simulink model "PubIfDecisionLM_MDL"  (R2020b)
settings: configuration reference "DspaceConfig" (kept outside this file)
PostLoadFcn:
  | if any(exist('dsrtsu_mdlpostloadfcn', 'file') ~= 0), dsrtsu_mdlpostloadfcn('Execute', bdroot); end
InitFcn:
  | , if any(exist('dsmpb_private', 'file') ~= 0), dsmpb_private('dsmpb_mdlclblib', 'Init', bdroot); end,
undefined symbols (not defined in the file or in its folder): OFM_OBJ_FUSIONTYPE_E, OFM_OBJ_MOVINGSTATE_E, OFM_OBJ_ORIENTATION_E, OFM_OBJ_TYPE_E, P_LM_Cyc, P_LM_EMLHistKapRcdBufSize, P_LM_EMLHistTrajBaseDis, P_LM_EMLHistTrajPNum, P_LM_EMLKapCorrMaxThre, P_LM_EMLMinKapThre, P_LM_EMLPathDisDiffThre, P_LM_EMLQuaFiltPar, P_LM_EMLTurnActKapThre, P_LM_EMLValidQuaThre, P_LM_FntPath1Disgap, P_LM_FntPath1MinDis, P_LM_FntPath1Timegap, P_LM_FntPath2Disgap, P_LM_FntPath2MinDis, P_LM_FntPath2Timegap, P_LM_FntPath3Disgap, P_LM_FntPath3MinDis, P_LM_FntPath3Timegap, P_LM_FusBLParFiltP, P_LM_FusEVDifC2Thre, P_LM_FusEVOPath1AllVSLDisThre, P_LM_FusEVOPath1AllVSLLostNumThre, P_LM_FusEVOPath1AllVSLQuaThre, P_LM_FusEVOPath1OTLFacNLC, P_LM_FusOTLQuaThre, P_LM_FusOTLSW, P_LM_FusParC0Index, P_LM_FusParC1Index, P_LM_FusParC2Index, P_LM_FusParC3Index, P_LM_FusVSLQuaThre, P_LM_FusVSLSW, P_LM_FusVSLValidSteerWheerAngThre, P_LM_FusVSLValidVxvThre, P_LM_LaneWidth, P_LM_OTLBufTPInfoEvaFactor, P_LM_OTLObjNum, P_LM_OTLObjSelectAgeThre, P_LM_OTLObjSelectDxAssessVx, P_LM_OTLObjSelectDxThre, P_LM_OTLObjSelectVxThre, P_LM_OTLObjSelectVyAssessDx, P_LM_OTLObjSelectVyThre, P_LM_OTLTrajPntBaseDis, P_LM_OTLTrajStdThre, P_LM_VSLAvailLineNum, P_LM_VSLBLSDiffThre, P_LM_VSLBLSDisRatio, P_LM_VSLFusBLParFiltP_C1, P_LM_VSLFusBLParFiltP_C2, P_LM_VSLFusBLParFiltP_C3, P_LM_VSLFusBLParFiltP_Quality, P_LM_VSLHistTrajBaseDis, P_LM_VSLHistTrajPNum, P_LM_VSLLCC0diff ... (+18)
libraries: simulink x145, LM_LIB x43
(part 11 of 24)

== system PubIfDecisionLM_MDL/Subsystem2/DIR/DrivingIntentionRecognition1/DIR_TurnDirProbCalc/DIR_TurnRightProbCalc/DIR_TurnRightProbCalcByCurveKap ==
  kapTraj : Inport
  1-D Lookup Table : Lookup_n-D  NumberOfTableDimensions=1  BreakpointsForDimension1=[0.01,0.014,0.018,0.022,0.026]  Table=[0,0.25,0.5,0.75,1]  InternalRulePriority=Speed  RndMeth=Simplest  InputSameDT=on
  Constant : Constant  Value=0.026  OutDataTypeStr=single
  Constant1 : Constant  OutDataTypeStr=single
  Constant2 : Constant  Value=0.01  OutDataTypeStr=single
  Constant3 : Constant  Value=0  OutDataTypeStr=single
  Constant4 : Constant  Value=-1  OutDataTypeStr=single
  Logical Operator : Logic  AllPortsSameDT=off  OutDataTypeStr=boolean
  Product : Product
  Relational Operator : RelationalOperator  OutDataTypeStr=boolean  RndMeth=Simplest
  Relational Operator1 : RelationalOperator  Operator=<  OutDataTypeStr=boolean  RndMeth=Simplest
  Relational Operator2 : RelationalOperator  OutDataTypeStr=boolean  RndMeth=Simplest
  Switch : Switch  Criteria=u2 ~= 0
  Switch1 : Switch  Criteria=u2 ~= 0
  DIR_TurnRightProbByKapTraj : Outport
  wires:
  kapTraj/1 -> Product/1
  Constant4/1 -> Product/2
  1-D Lookup Table/1 -> Switch1/1
  Switch/1 -> DIR_TurnRightProbByKapTraj/1  "LM_DIRTurnRightProbByKapTraj"
  Relational Operator1/1 -> Logical Operator/1
  Product/1 -> Relational Operator/1, Relational Operator1/1, Relational Operator2/1, 1-D Lookup Table/1
  Switch1/1 -> Switch/3
  Relational Operator/1 -> Switch/2
  Relational Operator2/1 -> Logical Operator/2
  Constant3/1 -> Switch1/3
  Constant/1 -> Relational Operator/2, Relational Operator1/2
  Constant1/1 -> Switch/1
  Logical Operator/1 -> Switch1/2
  Constant2/1 -> Relational Operator2/2

== system PubIfDecisionLM_MDL/Subsystem2/DIR/DrivingIntentionRecognition1/DIR_TurnDirProbCalc/DIR_TurnRightProbCalc/DIR_TurnRightProbCalcByPsiDtOpt ==
  PsiDtOpt : Inport
  1-D Lookup Table : Lookup_n-D  NumberOfTableDimensions=1  BreakpointsForDimension1=[0.11,0.15,0.19,0.23]  Table=[0,0.33,0.67,1]  InternalRulePriority=Speed  RndMeth=Simplest  InputSameDT=on
  Constant : Constant  Value=0.23  OutDataTypeStr=single
  Constant1 : Constant  OutDataTypeStr=single
  Constant2 : Constant  Value=0.11  OutDataTypeStr=single
  Constant3 : Constant  Value=0  OutDataTypeStr=single
  Constant4 : Constant  Value=-1  OutDataTypeStr=single
  Logical Operator : Logic  AllPortsSameDT=off  OutDataTypeStr=boolean
  Product : Product
  Relational Operator : RelationalOperator  OutDataTypeStr=boolean  RndMeth=Simplest
  Relational Operator1 : RelationalOperator  Operator=<  OutDataTypeStr=boolean  RndMeth=Simplest
  Relational Operator2 : RelationalOperator  OutDataTypeStr=boolean  RndMeth=Simplest
  Switch : Switch  Criteria=u2 ~= 0
  Switch1 : Switch  Criteria=u2 ~= 0
  DIR_TurnRightProbByPsiDtopt : Outport
  wires:
  Constant4/1 -> Product/2
  PsiDtOpt/1 -> Product/1
  1-D Lookup Table/1 -> Switch1/1
  Switch/1 -> DIR_TurnRightProbByPsiDtopt/1  "LM_DIRTurnRightProbByPsiDtopt"
  Switch1/1 -> Switch/3
  Constant3/1 -> Switch1/3
  Logical Operator/1 -> Switch1/2
  Relational Operator2/1 -> Logical Operator/2
  Relational Operator1/1 -> Logical Operator/1
  Constant2/1 -> Relational Operator2/2
  Constant1/1 -> Switch/1
  Relational Operator/1 -> Switch/2
  Constant/1 -> Relational Operator/2, Relational Operator1/2
  Product/1 -> Relational Operator/1, Relational Operator1/1, Relational Operator2/1, 1-D Lookup Table/1

== system PubIfDecisionLM_MDL/Subsystem2/DIR/DrivingIntentionRecognition1/DIR_TurnDirProbCalc/DIR_TurnRightProbCalc/DIR_TurnRightProbCalcBySteerWheelAng ==
  SteerWheelAngle : Inport
  SteerWheelAngleSign : Inport  Port=2
  1-D Lookup Table : Lookup_n-D  NumberOfTableDimensions=1  BreakpointsForDimension1=[85,90,95,100]  Table=[0,0.33,0.67,1]  InternalRulePriority=Speed  RndMeth=Simplest  InputSameDT=on
  Constant : Constant  Value=100  OutDataTypeStr=single
  Constant1 : Constant  OutDataTypeStr=single
  Constant2 : Constant  Value=85  OutDataTypeStr=single
  Constant3 : Constant  Value=0  OutDataTypeStr=single
  Constant4 : Constant  OutDataTypeStr=uint8
  Logical Operator : Logic  Inputs=3  AllPortsSameDT=off  OutDataTypeStr=boolean
  Logical Operator1 : Logic  AllPortsSameDT=off  OutDataTypeStr=boolean
  Relational Operator : RelationalOperator  OutDataTypeStr=boolean  RndMeth=Simplest
  Relational Operator1 : RelationalOperator  Operator=<  OutDataTypeStr=boolean  RndMeth=Simplest
  Relational Operator2 : RelationalOperator  OutDataTypeStr=boolean  RndMeth=Simplest
  Relational Operator3 : RelationalOperator  Operator===  OutDataTypeStr=boolean  RndMeth=Simplest
  Switch : Switch  Criteria=u2 ~= 0
  Switch1 : Switch  Criteria=u2 ~= 0
  DIR_TurnRightProbBySteerWheelAng : Outport
  wires:
  [SteerRightFlg] -> Logical Operator/3
  Logical Operator1/1 -> Switch/2
  Relational Operator3/1 -> Logical Operator1/1, [SteerRightFlg]
  Constant4/1 -> Relational Operator3/2
  SteerWheelAngleSign/1 -> Relational Operator3/1
  1-D Lookup Table/1 -> Switch1/1
  Switch1/1 -> Switch/3
  Constant3/1 -> Switch1/3
  Constant1/1 -> Switch/1
  Logical Operator/1 -> Switch1/2
  Constant2/1 -> Relational Operator2/2
  Relational Operator/1 -> Logical Operator1/2
  Relational Operator2/1 -> Logical Operator/2
  Constant/1 -> Relational Operator1/2, Relational Operator/2
  Relational Operator1/1 -> Logical Operator/1
  Switch/1 -> DIR_TurnRightProbBySteerWheelAng/1  "LM_DIRTurnRightProbBySteerWheelAng"
  SteerWheelAngle/1 -> Relational Operator/1, Relational Operator1/1, Relational Operator2/1, 1-D Lookup Table/1

== system PubIfDecisionLM_MDL/Subsystem2/DIR/DrivingIntentionRecognition1/DIR_TurnDirProbCalc/DIR_TurnRightProbCalc/DIR_TurnRightProbCalcByTurnLampSts ==
  RightTurnSWSts : Inport
  Constant : Constant  OutDataTypeStr=uint8
  Constant1 : Constant  OutDataTypeStr=single
  Constant2 : Constant  Value=0  OutDataTypeStr=single
  Relational Operator : RelationalOperator  Operator===  OutDataTypeStr=boolean  RndMeth=Simplest
  Switch : Switch  Criteria=u2 ~= 0
  DIR_TurnRightProbByTurnLampSts : Outport
  wires:
  Switch/1 -> DIR_TurnRightProbByTurnLampSts/1  "LM_DIRTurnRightProbByTurnLampSts"
  Constant2/1 -> Switch/3
  Constant1/1 -> Switch/1
  Relational Operator/1 -> Switch/2
  Constant/1 -> Relational Operator/2
  RightTurnSWSts/1 -> Relational Operator/1

== system PubIfDecisionLM_MDL/Subsystem2/DIR/DrivingIntentionRecognition1/DIR_TurnDirProbCalc/DIR_TurnRightProbCalc/DIR_TurnRightProbCalcByVehSpd ==
  vxvRefMs : Inport
  1-D Lookup Table : Lookup_n-D  NumberOfTableDimensions=1  BreakpointsForDimension1=[12,12.5,13,13.5,14]  Table=[1,0.75,0.5,0.25,0]  InternalRulePriority=Speed  RndMeth=Simplest  InputSameDT=on
  Constant : Constant  Value=12  OutDataTypeStr=single
  Constant1 : Constant  OutDataTypeStr=single
  Constant2 : Constant  Value=14  OutDataTypeStr=single
  Constant3 : Constant  Value=0  OutDataTypeStr=single
  Logical Operator : Logic  AllPortsSameDT=off  OutDataTypeStr=boolean
  Relational Operator : RelationalOperator  Operator=<=  OutDataTypeStr=boolean  RndMeth=Simplest
  Relational Operator1 : RelationalOperator  Operator=>  OutDataTypeStr=boolean  RndMeth=Simplest
  Relational Operator2 : RelationalOperator  Operator=<=  OutDataTypeStr=boolean  RndMeth=Simplest
  Switch : Switch  Criteria=u2 ~= 0
  Switch1 : Switch  Criteria=u2 ~= 0
  LM_DIRTurnRightProbByVehSpd : Outport
  wires:
  Switch/1 -> LM_DIRTurnRightProbByVehSpd/1  "LM_DIRTurnRightProbByVehSpd"
  Constant3/1 -> Switch1/3
  1-D Lookup Table/1 -> Switch1/1
  Switch1/1 -> Switch/3
  Logical Operator/1 -> Switch1/2
  Relational Operator2/1 -> Logical Operator/2
  Relational Operator1/1 -> Logical Operator/1
  Constant2/1 -> Relational Operator2/2
  Relational Operator/1 -> Switch/2
  Constant1/1 -> Switch/1
  Constant/1 -> Relational Operator1/2, Relational Operator/2
  vxvRefMs/1 -> Relational Operator/1, 1-D Lookup Table/1, Relational Operator1/1, Relational Operator2/1

== system PubIfDecisionLM_MDL/Subsystem2/LM_EML/LM_EMLFntPath1/LM_EMLKapAdjVal/LM_EMLMinKapWithin3Sec/If Action Subsystem ==
  kapTraj : Inport
  Action Port : ActionPort  ActionPortLabel=else
  LM_EMLMinKap : Outport
  wires:
  kapTraj/1 -> LM_EMLMinKap/1

== system PubIfDecisionLM_MDL/Subsystem2/LM_EML/LM_EMLFntPath1/LM_EMLKapAdjVal/LM_EMLMinKapWithin3Sec/If Action Subsystem1 ==
  LM_EMLKapBuf : Inport
  Action Port : ActionPort  ActionPortLabel=if(u1 ~= 0)
  Constant : Constant  Value=P_LM_EMLHistKapRcdBufSize  OutDataTypeStr=uint8
  LM_EMLKapBufMinValSearch : Subsystem  TreatAsAtomicUnit=on
  LM_EMLMinKap : Outport
  wires:
  LM_EMLKapBuf/1 -> LM_EMLKapBufMinValSearch/1(LM_EMLKapBuf)
  LM_EMLKapBufMinValSearch/1(LM_EMLMinKap) -> LM_EMLMinKap/1
  Constant/1 -> LM_EMLKapBufMinValSearch/2(P_LM_EMLHistKapRcdBufSize)

== system PubIfDecisionLM_MDL/Subsystem2/LM_EML/LM_EMLRearPath1/LM_EMLHistTrajCoordinateConvert/If Action Subsystem/For Each Subsystem ==
  LM_ComEVOffsetX : Inport
  LM_ComEVOffsetY : Inport  Port=2
  LM_ComEVOffsetAng : Inport  Port=3
  LM_EMLHistTrajVectXK1 : Inport  Port=4  Partition=on  PartitionDimension=1  PartitionWidth=1  PartitionOffset=0
  LM_EMLHistTrajVectYK1 : Inport  Port=5  Partition=on  PartitionDimension=1  PartitionWidth=1  PartitionOffset=0
  Add : Sum
  For Each : ForEach  DisableCoverage=on
  Product{,1..3} (4 alike) : Product
  Sin : Trigonometry
  Sin1 : Trigonometry  Operator=cos
  Subtract : Sum  Inputs=+-
  Subtract1 : Sum  Inputs=+-
  Subtract2 : Sum  Inputs=+-
  LM_EMLHistTrajVectXK1Adju : Outport  ConcatenationDimension=1
  LM_EMLHistTrajVectYK1Adju : Outport  Port=2  ConcatenationDimension=1
  wires:
  Product3/1 -> Add/2
  Product2/1 -> Add/1
  Subtract2/1 -> LM_EMLHistTrajVectXK1Adju/1  "LM_EMLHistTrajVectXK1Adju"
  Product1/1 -> Subtract2/2
  Product/1 -> Subtract2/1
  Sin/1 -> Product1/2, Product2/2
  Subtract1/1 -> Product1/1, Product3/1
  Sin1/1 -> Product/2, Product3/2
  LM_ComEVOffsetAng/1 -> Sin/1, Sin1/1
  Subtract/1 -> Product/1, Product2/1
  LM_ComEVOffsetY/1 -> Subtract1/2
  LM_EMLHistTrajVectYK1/1 -> Subtract1/1
  LM_ComEVOffsetX/1 -> Subtract/2
  LM_EMLHistTrajVectXK1/1 -> Subtract/1
  Add/1 -> LM_EMLHistTrajVectYK1Adju/1  "LM_EMLHistTrajVectYK1Adju"

== system PubIfDecisionLM_MDL/Subsystem2/LM_Fusion1/LM_FusBaseLineFilt/LM_FusBaseLineInfoFilt/LM_FusBLFntPath1InfoFilt/LM_FusBLPathQuliatyFilt ==
  note: P_LM_FusBLParFiltP
  LM_FusBLPathQuality : Inport
  LM_FusBLPathQualityK1 : Inport  Port=2
  Add11 : Sum
  Compare To Zero : simulink/Logic and Bit Operations/Compare To Zero  relop=~=  OutDataTypeStr=boolean
  Compare To Zero1 : simulink/Logic and Bit Operations/Compare To Zero  relop===  OutDataTypeStr=boolean
  Compare To Zero2 : simulink/Logic and Bit Operations/Compare To Zero  relop===  OutDataTypeStr=boolean
  Constant9 : Constant  Value=P_LM_FusBLParFiltP  OutDataTypeStr=single
  Data Type Conversion : DataTypeConversion  OutDataTypeStr=single
  Logical Operator : Logic  AllPortsSameDT=off  OutDataTypeStr=boolean
  MATLAB Function : MATLAB Function  TreatAsAtomicUnit=on
  Product16 : Product
  Subtract1 : Sum  Inputs=+-
  Switch1 : Switch  Criteria=u2 ~= 0
  Switch2 : Switch  Criteria=u2 ~= 0
  LM_FusBLPathQualityFilt : Outport
  wires:
  Compare To Zero/1 -> Logical Operator/1
  Subtract1/1 -> Product16/1
  Compare To Zero1/1 -> Logical Operator/2
  Constant9/1 -> Product16/2
  Product16/1 -> Add11/1
  LM_FusBLPathQualityK1/1 -> Data Type Conversion/1
  LM_FusBLPathQuality/1 -> Switch2/1, Compare To Zero/1, Switch1/1, Subtract1/1, Compare To Zero2/1  "LM_FusBLFntPath1C0"
  Add11/1 -> Switch1/3  "LM_FusBLPathC1"
  Logical Operator/1 -> Switch1/2
  Switch1/1 -> Switch2/3
  Compare To Zero2/1 -> Switch2/2
  Switch2/1 -> MATLAB Function/1(u1)
  MATLAB Function/1(y) -> LM_FusBLPathQualityFilt/1  "LM_FusBLPathQualityFilt"
  Data Type Conversion/1 -> Compare To Zero1/1, Subtract1/2, Add11/2, MATLAB Function/2(yk1)

== system PubIfDecisionLM_MDL/Subsystem2/LM_Fusion1/LM_FusBaseLineFilt/LM_FusBaseLineInfoFilt/LM_FusBLFntPath1InfoFilt/LM_Fus_BLFntPathC0Filt ==
  note: P_LM_FusBLParFiltP
  LM_FusBLPathC0 : Inport
  LM_FusBLPathQuality : Inport  Port=2
  LM_FusBLPathQualityK1 : Inport  Port=3
  LM_FusBLPathC0K1 : Inport  Port=4
  Add11 : Sum
  Compare To Zero : simulink/Logic and Bit Operations/Compare To Zero  relop=~=  OutDataTypeStr=boolean
  Compare To Zero1 : simulink/Logic and Bit Operations/Compare To Zero  relop===  OutDataTypeStr=boolean
  Constant9 : Constant  Value=P_LM_FusBLParFiltP  OutDataTypeStr=single
  Logical Operator : Logic  AllPortsSameDT=off  OutDataTypeStr=boolean
  MATLAB Function : MATLAB Function  TreatAsAtomicUnit=on
  Product16 : Product
  Subtract1 : Sum  Inputs=+-
  Switch1 : Switch  Criteria=u2 ~= 0
  LM_FusBLPathC0Filt : Outport
  wires:
  Compare To Zero/1 -> Logical Operator/1
  LM_FusBLPathQuality/1 -> Compare To Zero/1
  Product16/1 -> Add11/1
  Subtract1/1 -> Product16/1
  Constant9/1 -> Product16/2
  LM_FusBLPathC0/1 -> Switch1/1, Subtract1/1  "LM_FusBLFntPath1C0"
  Add11/1 -> Switch1/3  "LM_FusBLPathC1"
  LM_FusBLPathC0K1/1 -> Subtract1/2, Add11/2, MATLAB Function/2(yk1)
  Logical Operator/1 -> Switch1/2
  Switch1/1 -> MATLAB Function/1(u1)
  MATLAB Function/1(y) -> LM_FusBLPathC0Filt/1  "LM_FusBLPathC0Filt"
  LM_FusBLPathQualityK1/1 -> Compare To Zero1/1
  Compare To Zero1/1 -> Logical Operator/2

== system PubIfDecisionLM_MDL/Subsystem2/LM_Fusion1/LM_FusBaseLineFilt/LM_FusBaseLineInfoFilt/LM_FusBLFntPath1InfoFilt/LM_Fus_BLPath3C3Filt ==
  note: P_LM_FusBLParFiltP
  LM_FusBLPathQualityK1 : Inport
  LM_FusBLPathQuality : Inport  Port=2
  LM_FusBLPathC3BefFilt : Inport  Port=3
  LM_FusBLPathC3K1 : Inport  Port=4
  Add11 : Sum
  Compare To Zero : simulink/Logic and Bit Operations/Compare To Zero  relop=~=  OutDataTypeStr=boolean
  Compare To Zero1 : simulink/Logic and Bit Operations/Compare To Zero  relop===  OutDataTypeStr=boolean
  Constant9 : Constant  Value=P_LM_FusBLParFiltP  OutDataTypeStr=single
  Logical Operator : Logic  AllPortsSameDT=off  OutDataTypeStr=boolean
  MATLAB Function : MATLAB Function  TreatAsAtomicUnit=on
  Product16 : Product
  Subtract1 : Sum  Inputs=+-
  Switch1 : Switch  Criteria=u2 ~= 0
  LM_FusBLPathC3Filt : Outport
  wires:
  LM_FusBLPathQualityK1/1 -> Compare To Zero1/1
  Compare To Zero/1 -> Logical Operator/1
  LM_FusBLPathQuality/1 -> Compare To Zero/1
  Switch1/1 -> MATLAB Function/1(u1)
  MATLAB Function/1(y) -> LM_FusBLPathC3Filt/1  "LM_FusBLPathC3Filt"
  Subtract1/1 -> Product16/1
  Compare To Zero1/1 -> Logical Operator/2
  Constant9/1 -> Product16/2
  Product16/1 -> Add11/1
  LM_FusBLPathC3K1/1 -> Subtract1/2, Add11/2, MATLAB Function/2(yk1)
  LM_FusBLPathC3BefFilt/1 -> Switch1/1, Subtract1/1  "LM_FusBLFntPath1C0"
  Add11/1 -> Switch1/3  "LM_FusBLPathC1"
  Logical Operator/1 -> Switch1/2

== system PubIfDecisionLM_MDL/Subsystem2/LM_Fusion1/LM_FusBaseLineFilt/LM_FusBaseLineInfoFilt/LM_FusBLFntPath1InfoFilt/LM_Fus_BLPathC1Filt ==
  note: P_LM_FusBLParFiltP
  LM_FusBLPathQualityK1 : Inport
  LM_FusBLPathQuality : Inport  Port=2
  LM_FusBLPathC1BefFilt : Inport  Port=3
  LM_FusBLPathC1K1 : Inport  Port=4
  Add11 : Sum
  Compare To Zero : simulink/Logic and Bit Operations/Compare To Zero  relop=~=  OutDataTypeStr=boolean
  Compare To Zero1 : simulink/Logic and Bit Operations/Compare To Zero  relop===  OutDataTypeStr=boolean
  Constant9 : Constant  Value=P_LM_FusBLParFiltP  OutDataTypeStr=single
  Logical Operator : Logic  AllPortsSameDT=off  OutDataTypeStr=boolean
  MATLAB Function : MATLAB Function  TreatAsAtomicUnit=on
  Product16 : Product
  Subtract1 : Sum  Inputs=+-
  Switch1 : Switch  Criteria=u2 ~= 0
  LM_FusBLPathC1Filt : Outport
  wires:
  LM_FusBLPathQualityK1/1 -> Compare To Zero1/1
  Compare To Zero/1 -> Logical Operator/1
  LM_FusBLPathQuality/1 -> Compare To Zero/1
  Switch1/1 -> MATLAB Function/1(u1)
  MATLAB Function/1(y) -> LM_FusBLPathC1Filt/1  "LM_FusBLPathC1Filt"
  Subtract1/1 -> Product16/1
  Compare To Zero1/1 -> Logical Operator/2
  Constant9/1 -> Product16/2
  Product16/1 -> Add11/1
  LM_FusBLPathC1K1/1 -> Subtract1/2, Add11/2, MATLAB Function/2(yk1)
  LM_FusBLPathC1BefFilt/1 -> Switch1/1, Subtract1/1  "LM_FusBLFntPath1C0"
  Add11/1 -> Switch1/3  "LM_FusBLPathC1"
  Logical Operator/1 -> Switch1/2

== system PubIfDecisionLM_MDL/Subsystem2/LM_Fusion1/LM_FusBaseLineFilt/LM_FusBaseLineInfoFilt/LM_FusBLFntPath1InfoFilt/LM_Fus_BLPathC2Filt ==
  note: P_LM_FusBLParFiltP
  LM_FusBLPathQualityK1 : Inport
  LM_FusBLPathQuality : Inport  Port=2
  LM_FusBLPathC2BefFilt : Inport  Port=3
  LM_FusBLPathC2K1 : Inport  Port=4
  Add11 : Sum
  Compare To Zero : simulink/Logic and Bit Operations/Compare To Zero  relop=~=  OutDataTypeStr=boolean
  Compare To Zero1 : simulink/Logic and Bit Operations/Compare To Zero  relop===  OutDataTypeStr=boolean
  Constant9 : Constant  Value=P_LM_FusBLParFiltP  OutDataTypeStr=single
  Logical Operator : Logic  AllPortsSameDT=off  OutDataTypeStr=boolean
  MATLAB Function : MATLAB Function  TreatAsAtomicUnit=on
  Product16 : Product
  Subtract1 : Sum  Inputs=+-
  Switch1 : Switch  Criteria=u2 ~= 0
  LM_FusBLPathC2Filt : Outport
  wires:
  Logical Operator/1 -> Switch1/2
  Add11/1 -> Switch1/3  "LM_FusBLPathC1"
  LM_FusBLPathC2BefFilt/1 -> Subtract1/1, Switch1/1  "LM_FusBLFntPath1C0"
  LM_FusBLPathC2K1/1 -> MATLAB Function/2(yk1), Add11/2, Subtract1/2
  Product16/1 -> Add11/1
  Constant9/1 -> Product16/2
  Compare To Zero1/1 -> Logical Operator/2
  Subtract1/1 -> Product16/1
  MATLAB Function/1(y) -> LM_FusBLPathC2Filt/1  "LM_FusBLPathC2Filt"
  Switch1/1 -> MATLAB Function/1(u1)
  LM_FusBLPathQuality/1 -> Compare To Zero/1
  Compare To Zero/1 -> Logical Operator/1
  LM_FusBLPathQualityK1/1 -> Compare To Zero1/1

== system PubIfDecisionLM_MDL/Subsystem2/LM_Fusion1/LM_FusBaseLineInfoCalc/LM_FusBLFntPath1130/LM_EVOFFntPath2/LM_FusBLPathC0Calc ==
  LM_FusBLPathQuality : Inport
  LM_VSLPathP : Inport  Port=2
  LM_EMLPathP : Inport  Port=3
  LM_OTLPathP : Inport  Port=4
  LM_FusPathEMLK : Inport  Port=5
  LM_FusPathVSLK : Inport  Port=6
  LM_FusPathOTLK : Inport  Port=7
  Add : Sum
  Add5 : Sum
  Constant : Constant  Value=4  OutDataTypeStr=uint8
  Constant1 : Constant  Value=0  OutDataTypeStr=single
  Constant2 : Constant  Value=0  OutDataTypeStr=single
  Index Vector : MultiPortSwitch  Inputs=1
  Index Vector1 : MultiPortSwitch  Inputs=1
  Index Vector8 : MultiPortSwitch  Inputs=1
  Product : Product
  Product1 : Product
  Product10 : Product
  Relational Operator : RelationalOperator  Operator===  OutDataTypeStr=boolean  RndMeth=Simplest
  Switch : Switch  Criteria=u2 ~= 0
  LM_FusBLPathC0 : Outport
  wires:
  Relational Operator/1 -> Switch/2
  Switch/1 -> LM_FusBLPathC0/1  "LM_FusBLPathC0"
  LM_FusBLPathQuality/1 -> Relational Operator/1
  Constant2/1 -> Relational Operator/2
  Constant1/1 -> Switch/1
  Add/1 -> Add5/1  "LM_FusBLFntPath1C0"
  Product/1 -> Add/1
  Add5/1 -> Switch/3  "LM_FusBLFntPath1C0"
  Index Vector/1 -> Product/1
  Constant/1 -> Index Vector8/1, Index Vector1/1, Index Vector/1
  LM_FusPathOTLK/1 -> Product10/2
  LM_VSLPathP/1 -> Index Vector/2
  Product10/1 -> Add5/2
  LM_EMLPathP/1 -> Index Vector1/2
  LM_FusPathEMLK/1 -> Product1/2
  LM_OTLPathP/1 -> Index Vector8/2
  LM_FusPathVSLK/1 -> Product/2
  Index Vector8/1 -> Product10/1
  Index Vector1/1 -> Product1/1
  Product1/1 -> Add/2

== system PubIfDecisionLM_MDL/Subsystem2/LM_Fusion1/LM_FusBaseLineInfoCalc/LM_FusBLFntPath1130/LM_EVOFFntPath2/LM_FusBLPathC1Calc ==
  note: P_LM_FusBLParFiltP
  LM_FusBLPathQuality : Inport
  LM_VSLPathP : Inport  Port=2
  LM_EMLPathP : Inport  Port=3
  LM_OTLPathP : Inport  Port=4
  LM_FusPathEMLK : Inport  Port=5
  LM_FusPathVSLK : Inport  Port=6
  LM_FusPathOTLK : Inport  Port=7
  Add1 : Sum
  Add11 : Sum
  Add6 : Sum
  Constant1 : Constant  Value=3  OutDataTypeStr=uint8
  Constant2 : Constant  Value=0  OutDataTypeStr=single
  Constant3 : Constant  Value=0  OutDataTypeStr=single
  Constant9 : Constant  Value=P_LM_FusBLParFiltP  OutDataTypeStr=single
  Index Vector2 : MultiPortSwitch  Inputs=1
  Index Vector3 : MultiPortSwitch  Inputs=1
  Index Vector9 : MultiPortSwitch  Inputs=1
  Logical Operator : Logic  AllPortsSameDT=off  OutDataTypeStr=boolean
  Logical Operator1 : Logic  Operator=NOT  AllPortsSameDT=off  OutDataTypeStr=boolean
  MATLAB Function : MATLAB Function  TreatAsAtomicUnit=on
  Product{3..4,11,16} (4 alike) : Product
  Relational Operator : RelationalOperator  Operator===  OutDataTypeStr=boolean  RndMeth=Simplest
  Subtract1 : Sum  Inputs=+-
  Switch : Switch  Criteria=u2 ~= 0
  Switch1 : Switch  Criteria=u2 ~= 0
  Unit Delay1 : UnitDelay  SampleTime=-1  HasFrameUpgradeWarning=on
  Unit Delay2 : UnitDelay  SampleTime=-1  HasFrameUpgradeWarning=on
  LM_FusBLPathC1 : Outport
  wires:
  Switch/1 -> MATLAB Function/1(u1)  "LM_FusBLPathC1"
  Add11/1 -> Switch1/3  "LM_FusBLPathC1"
  Logical Operator/1 -> Switch1/2
  LM_FusBLPathQuality/1 -> Relational Operator/1
  Relational Operator/1 -> Logical Operator1/1, Switch/2, Unit Delay2/1
  Constant3/1 -> Relational Operator/2
  Constant2/1 -> Switch/1
  Logical Operator1/1 -> Logical Operator/1
  Unit Delay2/1 -> Logical Operator/2
  Switch1/1 -> Switch/3
  Add6/1 -> Subtract1/1, Switch1/1  "LM_FusBLFntPath1C0"
  Constant9/1 -> Product16/2
  Constant1/1 -> Index Vector9/1, Index Vector3/1, Index Vector2/1
  Subtract1/1 -> Product16/1
  Unit Delay1/1 -> Subtract1/2, Add11/2, MATLAB Function/2(yk1)
  Product3/1 -> Add1/1
  MATLAB Function/1(y) -> LM_FusBLPathC1/1, Unit Delay1/1  "LM_FusBLPathC1"
  LM_FusPathOTLK/1 -> Product11/2
  Add1/1 -> Add6/1  "LM_FusBLFntPath1C1"
  LM_VSLPathP/1 -> Index Vector2/2
  Product11/1 -> Add6/2
  LM_EMLPathP/1 -> Index Vector3/2
  Product16/1 -> Add11/1
  LM_FusPathEMLK/1 -> Product4/2
  LM_OTLPathP/1 -> Index Vector9/2
  LM_FusPathVSLK/1 -> Product3/2
  Index Vector9/1 -> Product11/1
  Product4/1 -> Add1/2
  Index Vector3/1 -> Product4/1
  Index Vector2/1 -> Product3/1

== system PubIfDecisionLM_MDL/Subsystem2/LM_Fusion1/LM_FusBaseLineInfoCalc/LM_FusBLFntPath1130/LM_EVOFFntPath2/LM_FusBLPathC2Calc ==
  note: P_LM_FusBLParFiltP
  LM_FusBLPathQuality : Inport
  LM_VSLPathP : Inport  Port=2
  LM_EMLPathP : Inport  Port=3
  LM_OTLPathP : Inport  Port=4
  LM_FusPathEMLK : Inport  Port=5
  LM_FusPathVSLK : Inport  Port=6
  LM_FusPathOTLK : Inport  Port=7
  Add12 : Sum
  Add2 : Sum
  Add7 : Sum
  Constant1 : Constant  Value=0  OutDataTypeStr=single
  Constant10 : Constant  Value=P_LM_FusBLParFiltP  OutDataTypeStr=single
  Constant2 : Constant  Value=2  OutDataTypeStr=uint8
  Constant3 : Constant  Value=0  OutDataTypeStr=single
  Index Vector10 : MultiPortSwitch  Inputs=1
  Index Vector4 : MultiPortSwitch  Inputs=1
  Index Vector5 : MultiPortSwitch  Inputs=1
  Logical Operator : Logic  AllPortsSameDT=off  OutDataTypeStr=boolean
  Logical Operator1 : Logic  Operator=NOT  AllPortsSameDT=off  OutDataTypeStr=boolean
  MATLAB Function : MATLAB Function  TreatAsAtomicUnit=on
  Product{2,5,12,17} (4 alike) : Product
  Relational Operator : RelationalOperator  Operator===  OutDataTypeStr=boolean  RndMeth=Simplest
  Subtract2 : Sum  Inputs=+-
  Switch : Switch  Criteria=u2 ~= 0
  Switch1 : Switch  Criteria=u2 ~= 0
  Unit Delay1 : UnitDelay  SampleTime=-1  HasFrameUpgradeWarning=on
  Unit Delay2 : UnitDelay  SampleTime=-1  HasFrameUpgradeWarning=on
  LM_FusBLPathC2 : Outport
  wires:
  Switch/1 -> MATLAB Function/1(u1)  "LM_FusBLPathC2"
  Unit Delay1/1 -> Logical Operator/2
  Switch1/1 -> Switch/3
  Constant1/1 -> Switch/1
  Logical Operator/1 -> Switch1/2
  Relational Operator/1 -> Logical Operator1/1, Switch/2, Unit Delay1/1
  Logical Operator1/1 -> Logical Operator/1
  Constant3/1 -> Relational Operator/2
  LM_FusBLPathQuality/1 -> Relational Operator/1
  Add12/1 -> Switch1/3  "LM_FusBLPathC1"
  Product17/1 -> Add12/1
  Subtract2/1 -> Product17/1
  Add7/1 -> Subtract2/1, Switch1/1  "LM_FusBLFntPath1C2"
  Constant10/1 -> Product17/2
  Constant2/1 -> Index Vector10/1, Index Vector5/1, Index Vector4/1
  Product12/1 -> Add7/2
  LM_FusPathEMLK/1 -> Product5/2
  Index Vector4/1 -> Product2/1
  Product5/1 -> Add2/2
  Add2/1 -> Add7/1  "LM_FusBLFntPath1C2"
  LM_FusPathOTLK/1 -> Product12/2
  LM_VSLPathP/1 -> Index Vector4/2
  Unit Delay2/1 -> Add12/2, Subtract2/2, MATLAB Function/2(yk1)
  LM_EMLPathP/1 -> Index Vector5/2
  LM_OTLPathP/1 -> Index Vector10/2
  LM_FusPathVSLK/1 -> Product2/2
  Index Vector10/1 -> Product12/1
  Index Vector5/1 -> Product5/1
  Product2/1 -> Add2/1
  MATLAB Function/1(y) -> LM_FusBLPathC2/1, Unit Delay2/1  "LM_FusBLPathC2"

== system PubIfDecisionLM_MDL/Subsystem2/LM_Fusion1/LM_FusBaseLineInfoCalc/LM_FusBLFntPath1130/LM_EVOFFntPath2/LM_FusBLPathC3Calc ==
  note: P_LM_FusBLParFiltP
  LM_FusBLPathQuality : Inport
  LM_VSLPathP : Inport  Port=2
  LM_EMLPathP : Inport  Port=3
  LM_OTLPathP : Inport  Port=4
  LM_FusPathEMLK : Inport  Port=5
  LM_FusPathVSLK : Inport  Port=6
  LM_FusPathOTLK : Inport  Port=7
  Add13 : Sum
  Add3 : Sum
  Add8 : Sum
  Constant1 : Constant  Value=0  OutDataTypeStr=single
  Constant11 : Constant  Value=P_LM_FusBLParFiltP  OutDataTypeStr=single
  Constant2 : Constant  Value=0  OutDataTypeStr=single
  Constant3 : Constant  OutDataTypeStr=uint8
  Index Vector11 : MultiPortSwitch  Inputs=1
  Index Vector6 : MultiPortSwitch  Inputs=1
  Index Vector7 : MultiPortSwitch  Inputs=1
  Logical Operator : Logic  AllPortsSameDT=off  OutDataTypeStr=boolean
  Logical Operator1 : Logic  Operator=NOT  AllPortsSameDT=off  OutDataTypeStr=boolean
  MATLAB Function : MATLAB Function  TreatAsAtomicUnit=on
  Product{6..7,13,18} (4 alike) : Product
  Relational Operator : RelationalOperator  Operator===  OutDataTypeStr=boolean  RndMeth=Simplest
  Subtract3 : Sum  Inputs=+-
  Switch : Switch  Criteria=u2 ~= 0
  Switch1 : Switch  Criteria=u2 ~= 0
  Unit Delay1 : UnitDelay  SampleTime=-1  HasFrameUpgradeWarning=on
  Unit Delay3 : UnitDelay  SampleTime=-1  HasFrameUpgradeWarning=on
  LM_FusBLPathC3 : Outport
  wires:
  Switch/1 -> MATLAB Function/1(u1)  "LM_FusBLPathC3"
  LM_FusBLPathQuality/1 -> Relational Operator/1
  Add13/1 -> Switch1/3  "LM_FusBLPathC1"
  Switch1/1 -> Switch/3
  Constant2/1 -> Relational Operator/2
  Logical Operator/1 -> Switch1/2
  Unit Delay1/1 -> Logical Operator/2
  Constant1/1 -> Switch/1
  Logical Operator1/1 -> Logical Operator/1
  Relational Operator/1 -> Logical Operator1/1, Switch/2, Unit Delay1/1
  Add8/1 -> Subtract3/1, Switch1/1
  Product6/1 -> Add3/1
  Index Vector6/1 -> Product6/1
  Add3/1 -> Add8/1  "LM_FusBLFntPath1C3"
  Product18/1 -> Add13/1
  Subtract3/1 -> Product18/1
  Index Vector7/1 -> Product7/1
  Constant11/1 -> Product18/2
  Index Vector11/1 -> Product13/1
  Product13/1 -> Add8/2
  Constant3/1 -> Index Vector11/1, Index Vector7/1, Index Vector6/1
  LM_FusPathEMLK/1 -> Product7/2
  Unit Delay3/1 -> Subtract3/2, Add13/2, MATLAB Function/2(yk1)
  LM_VSLPathP/1 -> Index Vector6/2
  LM_EMLPathP/1 -> Index Vector7/2
  LM_OTLPathP/1 -> Index Vector11/2
  Product7/1 -> Add3/2
  LM_FusPathVSLK/1 -> Product6/2
  MATLAB Function/1(y) -> LM_FusBLPathC3/1, Unit Delay3/1  "LM_FusBLPathC3"
  LM_FusPathOTLK/1 -> Product13/2

== system PubIfDecisionLM_MDL/Subsystem2/LM_Fusion1/LM_FusBaseLineInfoCalc/LM_FusBLFntPath1130/LM_EVOFFntPath3/LM_FusBLPathC0Calc ==
  LM_FusBLPathQuality : Inport
  LM_VSLPathP : Inport  Port=2
  LM_EMLPathP : Inport  Port=3
  LM_OTLPathP : Inport  Port=4
  LM_FusPathEMLK : Inport  Port=5
  LM_FusPathVSLK : Inport  Port=6
  LM_FusPathOTLK : Inport  Port=7
  Add : Sum
  Add5 : Sum
  Constant : Constant  Value=4  OutDataTypeStr=uint8
  Constant1 : Constant  Value=0  OutDataTypeStr=single
  Constant2 : Constant  Value=0  OutDataTypeStr=single
  Index Vector : MultiPortSwitch  Inputs=1
  Index Vector1 : MultiPortSwitch  Inputs=1
  Index Vector8 : MultiPortSwitch  Inputs=1
  Product : Product
  Product1 : Product
  Product10 : Product
  Relational Operator : RelationalOperator  Operator===  OutDataTypeStr=boolean  RndMeth=Simplest
  Switch : Switch  Criteria=u2 ~= 0
  LM_FusBLPathC0 : Outport
  wires:
  Relational Operator/1 -> Switch/2
  Switch/1 -> LM_FusBLPathC0/1  "LM_FusBLPathC0"
  LM_FusBLPathQuality/1 -> Relational Operator/1
  Constant2/1 -> Relational Operator/2
  Constant1/1 -> Switch/1
  Add/1 -> Add5/1  "LM_FusBLFntPath1C0"
  Product/1 -> Add/1
  Add5/1 -> Switch/3  "LM_FusBLFntPath1C0"
  Index Vector/1 -> Product/1
  Constant/1 -> Index Vector8/1, Index Vector1/1, Index Vector/1
  LM_FusPathOTLK/1 -> Product10/2
  LM_VSLPathP/1 -> Index Vector/2
  Product10/1 -> Add5/2
  LM_EMLPathP/1 -> Index Vector1/2
  LM_FusPathEMLK/1 -> Product1/2
  LM_OTLPathP/1 -> Index Vector8/2
  LM_FusPathVSLK/1 -> Product/2
  Index Vector8/1 -> Product10/1
  Index Vector1/1 -> Product1/1
  Product1/1 -> Add/2

== system PubIfDecisionLM_MDL/Subsystem2/LM_Fusion1/LM_FusBaseLineInfoCalc/LM_FusBLFntPath1130/LM_EVOFFntPath3/LM_FusBLPathC1Calc ==
  note: P_LM_FusBLParFiltP
  LM_FusBLPathQuality : Inport
  LM_VSLPathP : Inport  Port=2
  LM_EMLPathP : Inport  Port=3
  LM_OTLPathP : Inport  Port=4
  LM_FusPathEMLK : Inport  Port=5
  LM_FusPathVSLK : Inport  Port=6
  LM_FusPathOTLK : Inport  Port=7
  Add1 : Sum
  Add11 : Sum
  Add6 : Sum
  Constant1 : Constant  Value=3  OutDataTypeStr=uint8
  Constant2 : Constant  Value=0  OutDataTypeStr=single
  Constant3 : Constant  Value=0  OutDataTypeStr=single
  Constant9 : Constant  Value=P_LM_FusBLParFiltP  OutDataTypeStr=single
  Index Vector2 : MultiPortSwitch  Inputs=1
  Index Vector3 : MultiPortSwitch  Inputs=1
  Index Vector9 : MultiPortSwitch  Inputs=1
  Logical Operator : Logic  AllPortsSameDT=off  OutDataTypeStr=boolean
  Logical Operator1 : Logic  Operator=NOT  AllPortsSameDT=off  OutDataTypeStr=boolean
  MATLAB Function : MATLAB Function  TreatAsAtomicUnit=on
  Product{3..4,11,16} (4 alike) : Product
  Relational Operator : RelationalOperator  Operator===  OutDataTypeStr=boolean  RndMeth=Simplest
  Subtract1 : Sum  Inputs=+-
  Switch : Switch  Criteria=u2 ~= 0
  Switch1 : Switch  Criteria=u2 ~= 0
  Unit Delay1 : UnitDelay  SampleTime=-1  HasFrameUpgradeWarning=on
  Unit Delay2 : UnitDelay  SampleTime=-1  HasFrameUpgradeWarning=on
  LM_FusBLPathC1 : Outport
  wires:
  Switch/1 -> MATLAB Function/1(u1)  "LM_FusBLPathC1"
  Add11/1 -> Switch1/3  "LM_FusBLPathC1"
  Logical Operator/1 -> Switch1/2
  LM_FusBLPathQuality/1 -> Relational Operator/1
  Relational Operator/1 -> Logical Operator1/1, Switch/2, Unit Delay2/1
  Constant3/1 -> Relational Operator/2
  Constant2/1 -> Switch/1
  Logical Operator1/1 -> Logical Operator/1
  Unit Delay2/1 -> Logical Operator/2
  Switch1/1 -> Switch/3
  Add6/1 -> Subtract1/1, Switch1/1  "LM_FusBLFntPath1C0"
  Constant9/1 -> Product16/2
  Constant1/1 -> Index Vector9/1, Index Vector3/1, Index Vector2/1
  Subtract1/1 -> Product16/1
  Unit Delay1/1 -> Subtract1/2, Add11/2, MATLAB Function/2(yk1)
  Product3/1 -> Add1/1
  MATLAB Function/1(y) -> LM_FusBLPathC1/1, Unit Delay1/1  "LM_FusBLPathC1"
  LM_FusPathOTLK/1 -> Product11/2
  Add1/1 -> Add6/1  "LM_FusBLFntPath1C1"
  LM_VSLPathP/1 -> Index Vector2/2
  Product11/1 -> Add6/2
  LM_EMLPathP/1 -> Index Vector3/2
  Product16/1 -> Add11/1
  LM_FusPathEMLK/1 -> Product4/2
  LM_OTLPathP/1 -> Index Vector9/2
  LM_FusPathVSLK/1 -> Product3/2
  Index Vector9/1 -> Product11/1
  Product4/1 -> Add1/2
  Index Vector3/1 -> Product4/1
  Index Vector2/1 -> Product3/1

== system PubIfDecisionLM_MDL/Subsystem2/LM_Fusion1/LM_FusBaseLineInfoCalc/LM_FusBLFntPath1130/LM_EVOFFntPath3/LM_FusBLPathC2Calc ==
  note: P_LM_FusBLParFiltP
  LM_FusBLPathQuality : Inport
  LM_VSLPathP : Inport  Port=2
  LM_EMLPathP : Inport  Port=3
  LM_OTLPathP : Inport  Port=4
  LM_FusPathEMLK : Inport  Port=5
  LM_FusPathVSLK : Inport  Port=6
  LM_FusPathOTLK : Inport  Port=7
  Add12 : Sum
  Add2 : Sum
  Add7 : Sum
  Constant1 : Constant  Value=0  OutDataTypeStr=single
  Constant10 : Constant  Value=P_LM_FusBLParFiltP  OutDataTypeStr=single
  Constant2 : Constant  Value=2  OutDataTypeStr=uint8
  Constant3 : Constant  Value=0  OutDataTypeStr=single
  Index Vector10 : MultiPortSwitch  Inputs=1
  Index Vector4 : MultiPortSwitch  Inputs=1
  Index Vector5 : MultiPortSwitch  Inputs=1
  Logical Operator : Logic  AllPortsSameDT=off  OutDataTypeStr=boolean
  Logical Operator1 : Logic  Operator=NOT  AllPortsSameDT=off  OutDataTypeStr=boolean
  MATLAB Function : MATLAB Function  TreatAsAtomicUnit=on
  Product{2,5,12,17} (4 alike) : Product
  Relational Operator : RelationalOperator  Operator===  OutDataTypeStr=boolean  RndMeth=Simplest
  Subtract2 : Sum  Inputs=+-
  Switch : Switch  Criteria=u2 ~= 0
  Switch1 : Switch  Criteria=u2 ~= 0
  Unit Delay1 : UnitDelay  SampleTime=-1  HasFrameUpgradeWarning=on
  Unit Delay2 : UnitDelay  SampleTime=-1  HasFrameUpgradeWarning=on
  LM_FusBLPathC2 : Outport
  wires:
  Switch/1 -> MATLAB Function/1(u1)  "LM_FusBLPathC2"
  Unit Delay1/1 -> Logical Operator/2
  Switch1/1 -> Switch/3
  Constant1/1 -> Switch/1
  Logical Operator/1 -> Switch1/2
  Relational Operator/1 -> Logical Operator1/1, Switch/2, Unit Delay1/1
  Logical Operator1/1 -> Logical Operator/1
  Constant3/1 -> Relational Operator/2
  LM_FusBLPathQuality/1 -> Relational Operator/1
  Add12/1 -> Switch1/3  "LM_FusBLPathC1"
  Product17/1 -> Add12/1
  Subtract2/1 -> Product17/1
  Add7/1 -> Subtract2/1, Switch1/1  "LM_FusBLFntPath1C2"
  Constant10/1 -> Product17/2
  Constant2/1 -> Index Vector10/1, Index Vector5/1, Index Vector4/1
  Product12/1 -> Add7/2
  LM_FusPathEMLK/1 -> Product5/2
  Index Vector4/1 -> Product2/1
  Product5/1 -> Add2/2
  Add2/1 -> Add7/1  "LM_FusBLFntPath1C2"
  LM_FusPathOTLK/1 -> Product12/2
  LM_VSLPathP/1 -> Index Vector4/2
  Unit Delay2/1 -> Add12/2, Subtract2/2, MATLAB Function/2(yk1)
  LM_EMLPathP/1 -> Index Vector5/2
  LM_OTLPathP/1 -> Index Vector10/2
  LM_FusPathVSLK/1 -> Product2/2
  Index Vector10/1 -> Product12/1
  Index Vector5/1 -> Product5/1
  Product2/1 -> Add2/1
  MATLAB Function/1(y) -> LM_FusBLPathC2/1, Unit Delay2/1  "LM_FusBLPathC2"

== system PubIfDecisionLM_MDL/Subsystem2/LM_Fusion1/LM_FusBaseLineInfoCalc/LM_FusBLFntPath1130/LM_EVOFFntPath3/LM_FusBLPathC3Calc ==
  note: P_LM_FusBLParFiltP
  LM_FusBLPathQuality : Inport
  LM_VSLPathP : Inport  Port=2
  LM_EMLPathP : Inport  Port=3
  LM_OTLPathP : Inport  Port=4
  LM_FusPathEMLK : Inport  Port=5
  LM_FusPathVSLK : Inport  Port=6
  LM_FusPathOTLK : Inport  Port=7
  Add13 : Sum
  Add3 : Sum
  Add8 : Sum
  Constant1 : Constant  Value=0  OutDataTypeStr=single
  Constant11 : Constant  Value=P_LM_FusBLParFiltP  OutDataTypeStr=single
  Constant2 : Constant  Value=0  OutDataTypeStr=single
  Constant3 : Constant  OutDataTypeStr=uint8
  Index Vector11 : MultiPortSwitch  Inputs=1
  Index Vector6 : MultiPortSwitch  Inputs=1
  Index Vector7 : MultiPortSwitch  Inputs=1
  Logical Operator : Logic  AllPortsSameDT=off  OutDataTypeStr=boolean
  Logical Operator1 : Logic  Operator=NOT  AllPortsSameDT=off  OutDataTypeStr=boolean
  MATLAB Function : MATLAB Function  TreatAsAtomicUnit=on
  Product{6..7,13,18} (4 alike) : Product
  Relational Operator : RelationalOperator  Operator===  OutDataTypeStr=boolean  RndMeth=Simplest
  Subtract3 : Sum  Inputs=+-
  Switch : Switch  Criteria=u2 ~= 0
  Switch1 : Switch  Criteria=u2 ~= 0
  Unit Delay1 : UnitDelay  SampleTime=-1  HasFrameUpgradeWarning=on
  Unit Delay3 : UnitDelay  SampleTime=-1  HasFrameUpgradeWarning=on
  LM_FusBLPathC3 : Outport
  wires:
  Switch/1 -> MATLAB Function/1(u1)  "LM_FusBLPathC3"
  LM_FusBLPathQuality/1 -> Relational Operator/1
  Add13/1 -> Switch1/3  "LM_FusBLPathC1"
  Switch1/1 -> Switch/3
  Constant2/1 -> Relational Operator/2
  Logical Operator/1 -> Switch1/2
  Unit Delay1/1 -> Logical Operator/2
  Constant1/1 -> Switch/1
  Logical Operator1/1 -> Logical Operator/1
  Relational Operator/1 -> Logical Operator1/1, Switch/2, Unit Delay1/1
  Add8/1 -> Subtract3/1, Switch1/1
  Product6/1 -> Add3/1
  Index Vector6/1 -> Product6/1
  Add3/1 -> Add8/1  "LM_FusBLFntPath1C3"
  Product18/1 -> Add13/1
  Subtract3/1 -> Product18/1
  Index Vector7/1 -> Product7/1
  Constant11/1 -> Product18/2
  Index Vector11/1 -> Product13/1
  Product13/1 -> Add8/2
  Constant3/1 -> Index Vector11/1, Index Vector7/1, Index Vector6/1
  LM_FusPathEMLK/1 -> Product7/2
  Unit Delay3/1 -> Subtract3/2, Add13/2, MATLAB Function/2(yk1)
  LM_VSLPathP/1 -> Index Vector6/2
  LM_EMLPathP/1 -> Index Vector7/2
  LM_OTLPathP/1 -> Index Vector11/2
  Product7/1 -> Add3/2
  LM_FusPathVSLK/1 -> Product6/2
  MATLAB Function/1(y) -> LM_FusBLPathC3/1, Unit Delay3/1  "LM_FusBLPathC3"
  LM_FusPathOTLK/1 -> Product13/2

== system PubIfDecisionLM_MDL/Subsystem2/LM_Fusion1/LM_FusRatioCalc/LM_Fusion_EMLOnly/LM_FusEMLAndVSLRatioCalc/LM_Fusion_RearPathK ==
  Constant{,2,4..5} (4 alike) : Constant  Value=0  OutDataTypeStr=single
  Constant1 : Constant  OutDataTypeStr=single
  Constant3 : Constant  OutDataTypeStr=single
  LM_FusRearPath1VSLK : Outport
  LM_FusRearPath2VSLK : Outport  Port=2
  LM_FusRearPath3VSLK : Outport  Port=3
  LM_FusRearPath1EMLK : Outport  Port=4
  LM_FusRearPath2EMLK : Outport  Port=5
  LM_FusRearPath3EMLK : Outport  Port=6
  wires:
  Constant/1 -> LM_FusRearPath1VSLK/1  "LM_FusRearPath1VSLK"
  Constant1/1 -> LM_FusRearPath1EMLK/1  "LM_FusRearPath1EMLK"
  Constant2/1 -> LM_FusRearPath2VSLK/1  "LM_FusRearPath2VSLK"
  Constant5/1 -> LM_FusRearPath3EMLK/1  "LM_FusRearPath3EMLK"
  Constant4/1 -> LM_FusRearPath3VSLK/1  "LM_FusRearPath3VSLK"
  Constant3/1 -> LM_FusRearPath2EMLK/1  "LM_FusRearPath2EMLK"

== system PubIfDecisionLM_MDL/Subsystem2/LM_Fusion1/LM_FusRatioCalc/LM_Fusion_EO/LM_FusEVORatioCalc/LM_Fusion_FntPathK ==
  LM_EMLFntPath1Quality : Inport
  LM_EMLFntPath2Quality : Inport  Port=2
  LM_EMLFntPath3Quality : Inport  Port=3
  LM_OTLFntPath1Qulity : Inport  Port=4
  LM_OTLFntPath2Qulity : Inport  Port=5
  LM_OTLFntPath3Qulity : Inport  Port=6
  vxvRefMs : Inport  Port=7
  DIR_TurnLeftValid : Inport  Port=8
  DIR_TurnRightValid : Inport  Port=9
  DIR_LC2LeValid : Inport  Port=10
  DIR_LC2RigValid : Inport  Port=11
  LM_FusEOFntPath1 : Subsystem
  LM_FusEOFntPath2 : Subsystem
  LM_FusEOFntPath3 : Subsystem
  LM_FusEOFusTypeCalc : Subsystem
  LM_FusEOFntPath1EMLK : Outport
  LM_FusEOFntPath1VSLK : Outport  Port=2
  LM_FusEOFntPath1OTLK : Outport  Port=3
  LM_FusEOFntPath1RELK : Outport  Port=4
  LM_FusEOFntPath1MALK : Outport  Port=5
  LM_FusEOFntPath2EMLK : Outport  Port=6
  LM_FusEOFntPath2VSLK : Outport  Port=7
  LM_FusEOFntPath2OTLK : Outport  Port=8
  LM_FusEOFntPath2RELK : Outport  Port=9
  LM_FusEOFntPath2MALK : Outport  Port=10
  LM_FusEOFntPath3EMLK : Outport  Port=11
  LM_FusEOFntPath3VSLK : Outport  Port=12
  LM_FusEOFntPath3OTLK : Outport  Port=13
  LM_FusEOFntPath3RELK : Outport  Port=14
  LM_FusEOFntPath3MALK : Outport  Port=15
  wires:
  LM_FusEOFntPath3/3(LM_FusEOFntPath3OTLK) -> LM_FusEOFntPath3OTLK/1
  LM_FusEOFntPath3/2(LM_FusEOFntPath3VSLK) -> LM_FusEOFntPath3VSLK/1
  LM_FusEOFntPath3/1(LM_FusEOFntPath3EMLK) -> LM_FusEOFntPath3EMLK/1
  LM_FusEOFntPath2/3(LM_FusEOFntPath2OTLK) -> LM_FusEOFntPath2OTLK/1
  LM_FusEOFntPath2/2(LM_FusEOFntPath2VSLK) -> LM_FusEOFntPath2VSLK/1
  LM_FusEOFntPath2/1(LM_FusEOFntPath2EMLK) -> LM_FusEOFntPath2EMLK/1
  LM_FusEOFntPath1/3(LM_FusEOFntPath1OTLK) -> LM_FusEOFntPath1OTLK/1
  LM_FusEOFntPath1/2(LM_FusEOFntPath1VSLK) -> LM_FusEOFntPath1VSLK/1
  LM_FusEOFntPath1/1(LM_FusEOFntPath1EMLK) -> LM_FusEOFntPath1EMLK/1
  LM_OTLFntPath3Qulity/1 -> LM_FusEOFntPath3/3(LM_OTLFntPath3Qulity)
  LM_EMLFntPath3Quality/1 -> LM_FusEOFntPath3/2(LM_EMLFntPath3Quality)
  LM_OTLFntPath2Qulity/1 -> LM_FusEOFntPath2/4(LM_OTLFntPath2Qulity)
  LM_EMLFntPath2Quality/1 -> LM_FusEOFntPath2/3(LM_EMLFntPath2Quality)
  vxvRefMs/1 -> LM_FusEOFntPath2/1(vxvRefMs), LM_FusEOFntPath1/1(vxvRefMs)
  LM_OTLFntPath1Qulity/1 -> LM_FusEOFntPath1/3(LM_OTLFntPath1Qulity)
  LM_EMLFntPath1Quality/1 -> LM_FusEOFntPath1/2(LM_EMLFntPath1Quality)
  LM_FusEOFntPath1/4(LM_FusEOFntPath1RELK) -> LM_FusEOFntPath1RELK/1
  LM_FusEOFntPath1/5(LM_FusEOFntPath1MALK) -> LM_FusEOFntPath1MALK/1
  LM_FusEOFntPath2/4(LM_FusEOFntPath2RELK) -> LM_FusEOFntPath2RELK/1
  LM_FusEOFntPath2/5(LM_FusEOFntPath2MALK) -> LM_FusEOFntPath2MALK/1
  LM_FusEOFntPath3/4(LM_FusEOFntPath3RELK) -> LM_FusEOFntPath3RELK/1
  LM_FusEOFntPath3/5(LM_FusEOFntPath3MALK) -> LM_FusEOFntPath3MALK/1
  LM_FusEOFusTypeCalc/1(LM_FusEOFusType) -> LM_FusEOFntPath3/1(LM_FusEOFusType), LM_FusEOFntPath2/2(LM_FusEOFusType), LM_FusEOFntPath1/4(LM_FusEOFusType)
  DIR_TurnLeftValid/1 -> LM_FusEOFusTypeCalc/1(DIR_TurnLeftValid)
  DIR_TurnRightValid/1 -> LM_FusEOFusTypeCalc/2(DIR_TurnRightValid)
  DIR_LC2LeValid/1 -> LM_FusEOFusTypeCalc/3(DIR_LC2LeValid)
  DIR_LC2RigValid/1 -> LM_FusEOFusTypeCalc/4(DIR_LC2RigValid)

== system PubIfDecisionLM_MDL/Subsystem2/LM_Fusion1/LM_FusRatioCalc/LM_Fusion_EO/LM_FusEVORatioCalc/LM_Fusion_RearPathK ==
  Constant{,1..5} (6 alike) : Constant  Value=0  OutDataTypeStr=single
  LM_FusRearPath1VSLK : Outport
  LM_FusRearPath2VSLK : Outport  Port=2
  LM_FusRearPath3VSLK : Outport  Port=3
  LM_FusRearPath1EMLK : Outport  Port=4
  LM_FusRearPath2EMLK : Outport  Port=5
  LM_FusRearPath3EMLK : Outport  Port=6
  wires:
  Constant/1 -> LM_FusRearPath1VSLK/1  "LM_FusRearPath1VSLK"
  Constant1/1 -> LM_FusRearPath1EMLK/1  "LM_FusRearPath1EMLK"
  Constant2/1 -> LM_FusRearPath2VSLK/1  "LM_FusRearPath2VSLK"
  Constant5/1 -> LM_FusRearPath3EMLK/1  "LM_FusRearPath3EMLK"
  Constant4/1 -> LM_FusRearPath3VSLK/1  "LM_FusRearPath3VSLK"
  Constant3/1 -> LM_FusRearPath2EMLK/1  "LM_FusRearPath2EMLK"

== system PubIfDecisionLM_MDL/Subsystem2/LM_Fusion1/LM_FusRatioCalc/LM_Fusion_EV/LM_FusBaseLineC0Info/If Action Subsystem ==
  LM_EMLLLC0Adju : Inport
  LM_EMLLRC0Adju : Inport  Port=2
  LM_EMLRLC0Adju : Inport  Port=3
  LM_EMLRRC0Adju : Inport  Port=4
  Action Port : ActionPort  ActionPortLabel=if(u1 ~= 0)
  Signal Conversion{,1..3} (4 alike) : SignalConversion  OverrideOpt=off
  LM_LLC0 : Outport
  LM_LRC0 : Outport  Port=2
  LM_RLC0 : Outport  Port=3
  LM_RRC0 : Outport  Port=4
  wires:
  LM_EMLRRC0Adju/1 -> Signal Conversion3/1
  LM_EMLLLC0Adju/1 -> Signal Conversion/1
  LM_EMLLRC0Adju/1 -> Signal Conversion1/1
  Signal Conversion3/1 -> LM_RRC0/1  "LM_RRC0"
  LM_EMLRLC0Adju/1 -> Signal Conversion2/1
  Signal Conversion1/1 -> LM_LRC0/1  "LM_LRC0"
  Signal Conversion2/1 -> LM_RLC0/1  "LM_RLC0"
  Signal Conversion/1 -> LM_LLC0/1  "LM_LLC0"

== system PubIfDecisionLM_MDL/Subsystem2/LM_Fusion1/LM_FusRatioCalc/LM_Fusion_EV/LM_FusBaseLineC0Info/If Action Subsystem1 ==
  LM_VSLLLC0Adju : Inport
  LM_VSLLRC0Adju : Inport  Port=2
  LM_VSLRLC0Adju : Inport  Port=3
  LM_VSLRRC0Adju : Inport  Port=4
  Action Port : ActionPort  ActionPortLabel=else
  Signal Conversion{,1..3} (4 alike) : SignalConversion  OverrideOpt=off
  LM_LLC0 : Outport
  LM_LRC0 : Outport  Port=2
  LM_RLC0 : Outport  Port=3
  LM_RRC0 : Outport  Port=4
  wires:
  LM_VSLRRC0Adju/1 -> Signal Conversion3/1
  LM_VSLLLC0Adju/1 -> Signal Conversion/1
  LM_VSLLRC0Adju/1 -> Signal Conversion1/1
  Signal Conversion3/1 -> LM_RRC0/1  "LM_RRC0"
  LM_VSLRLC0Adju/1 -> Signal Conversion2/1
  Signal Conversion1/1 -> LM_LRC0/1  "LM_LRC0"
  Signal Conversion2/1 -> LM_RLC0/1  "LM_RLC0"
  Signal Conversion/1 -> LM_LLC0/1  "LM_LLC0"

== system PubIfDecisionLM_MDL/Subsystem2/LM_Fusion1/LM_FusRatioCalc/LM_Fusion_EV/LM_FusEMLAndVSLRatioCalc/LM_Fusion_FntPathK ==
  LM_VSLFntPath1Quality : Inport
  LM_VSLFntPath2Quality : Inport  Port=2
  LM_VSLFntPath3Quality : Inport  Port=3
  LM_VSLFntPath1P : Inport  Port=4
  LM_VSLBaseDis : Inport  Port=5
  LM_EMLFntPath1Quality : Inport  Port=6
  LM_EMLFntPath2Quality : Inport  Port=7
  LM_EMLFntPath3Quality : Inport  Port=8
  LM_EMLFntPath1P : Inport  Port=9
  LM_ComLineLostNum : Inport  Port=10
  DIR_TurnLeftValid : Inport  Port=11
  DIR_TurnRightValid : Inport  Port=12
  DIR_LC2LeValid : Inport  Port=13
  DIR_LC2RigValid : Inport  Port=14
  vxvRefMs : Inport  Port=15
  Constant{,1..8} (9 alike) : Constant  Value=0  OutDataTypeStr=single
  LM_EVF_DeviationCalc : Subsystem
  LM_Fusion_VSL_EMLPath1KCalc1 : MATLAB Function  TreatAsAtomicUnit=on
  LM_FusEVFntPath1EMLK : Outport
  LM_FusEVFntPath1VSLK : Outport  Port=2
  LM_FusEVFntPath1OTLK : Outport  Port=3
  LM_FusEVFntPath1RELK : Outport  Port=4
  LM_FusEVFntPath1MALK : Outport  Port=5
  LM_FusEVFntPath2EMLK : Outport  Port=6
  LM_FusEVFntPath2VSLK : Outport  Port=7
  LM_FusEVFntPath2OTLK : Outport  Port=8
  LM_FusEVFntPath2RELK : Outport  Port=9
  LM_FusEVFntPath2MALK : Outport  Port=10
  LM_FusEVFntPath3EMLK : Outport  Port=11
  LM_FusEVFntPath3VSLK : Outport  Port=12
  LM_FusEVFntPath3OTLK : Outport  Port=13
  LM_FusEVFntPath3RELK : Outport  Port=14
  LM_FusEVFntPath3MALK : Outport  Port=15
  wires:
  LM_Fusion_VSL_EMLPath1KCalc1/3(LM_FusEVFntPath3VSLK) -> LM_FusEVFntPath3VSLK/1
  LM_Fusion_VSL_EMLPath1KCalc1/6(LM_FusEVFntPath3EMLK) -> LM_FusEVFntPath3EMLK/1
  LM_EMLFntPath3Quality/1 -> LM_Fusion_VSL_EMLPath1KCalc1/6(LM_EMLFntPath3Quality)
  LM_VSLFntPath3Quality/1 -> LM_Fusion_VSL_EMLPath1KCalc1/3(LM_VSLFntPath3Quality)
  LM_Fusion_VSL_EMLPath1KCalc1/2(LM_FusEVFntPath2VSLK) -> LM_FusEVFntPath2VSLK/1
  LM_Fusion_VSL_EMLPath1KCalc1/5(LM_FusEVFntPath2EMLK) -> LM_FusEVFntPath2EMLK/1
  LM_Fusion_VSL_EMLPath1KCalc1/1(LM_FusEVFntPath1VSLK) -> LM_FusEVFntPath1VSLK/1
  LM_EMLFntPath2Quality/1 -> LM_Fusion_VSL_EMLPath1KCalc1/5(LM_EMLFntPath2Quality)
  LM_VSLFntPath2Quality/1 -> LM_Fusion_VSL_EMLPath1KCalc1/2(LM_VSLFntPath2Quality)
  LM_EVF_DeviationCalc/1(LM_FusEVdiffValid) -> LM_Fusion_VSL_EMLPath1KCalc1/7(LM_FusEVdiffValid)
  LM_VSLFntPath1Quality/1 -> LM_Fusion_VSL_EMLPath1KCalc1/1(LM_VSLFntPath1Quality)
  LM_Fusion_VSL_EMLPath1KCalc1/4(LM_FusEVFntPath1EMLK) -> LM_FusEVFntPath1EMLK/1
  LM_EMLFntPath1Quality/1 -> LM_Fusion_VSL_EMLPath1KCalc1/4(LM_EMLFntPath1Quality)
  LM_ComLineLostNum/1 -> LM_Fusion_VSL_EMLPath1KCalc1/8(LM_ComLineLostNum)
  LM_VSLBaseDis/1 -> LM_Fusion_VSL_EMLPath1KCalc1/9(LM_VSLBaseDis)
  Constant/1 -> LM_FusEVFntPath1OTLK/1
  Constant1/1 -> LM_FusEVFntPath2OTLK/1
  Constant2/1 -> LM_FusEVFntPath3OTLK/1
  Constant5/1 -> LM_FusEVFntPath3RELK/1
  Constant4/1 -> LM_FusEVFntPath2RELK/1
  Constant3/1 -> LM_FusEVFntPath1RELK/1
  Constant6/1 -> LM_FusEVFntPath1MALK/1
  Constant7/1 -> LM_FusEVFntPath2MALK/1
  Constant8/1 -> LM_FusEVFntPath3MALK/1
  DIR_TurnLeftValid/1 -> LM_Fusion_VSL_EMLPath1KCalc1/10(DIR_TurnLeftValid)
  DIR_TurnRightValid/1 -> LM_Fusion_VSL_EMLPath1KCalc1/11(DIR_TurnRightValid)
  DIR_LC2LeValid/1 -> LM_Fusion_VSL_EMLPath1KCalc1/12(DIR_LC2LeValid)
  DIR_LC2RigValid/1 -> LM_Fusion_VSL_EMLPath1KCalc1/13(DIR_LC2RigValid)
  LM_EMLFntPath1P/1 -> LM_EVF_DeviationCalc/2(LM_EMLFntPath1P)
  LM_VSLFntPath1P/1 -> LM_EVF_DeviationCalc/1(LM_VSLFntPath1P)
  vxvRefMs/1 -> LM_Fusion_VSL_EMLPath1KCalc1/14(vxvRefMs)

== system PubIfDecisionLM_MDL/Subsystem2/LM_Fusion1/LM_FusRatioCalc/LM_Fusion_EV/LM_FusEMLAndVSLRatioCalc/LM_Fusion_RearPathK ==
  Constant{,1..5} (6 alike) : Constant  Value=0  OutDataTypeStr=single
  LM_FusRearPath1VSLK : Outport
  LM_FusRearPath2VSLK : Outport  Port=2
  LM_FusRearPath3VSLK : Outport  Port=3
  LM_FusRearPath1EMLK : Outport  Port=4
  LM_FusRearPath2EMLK : Outport  Port=5
  LM_FusRearPath3EMLK : Outport  Port=6
  wires:
  Constant3/1 -> LM_FusRearPath2EMLK/1  "LM_FusRearPath2EMLK"
  Constant4/1 -> LM_FusRearPath3VSLK/1  "LM_FusRearPath3VSLK"
  Constant5/1 -> LM_FusRearPath3EMLK/1  "LM_FusRearPath3EMLK"
  Constant2/1 -> LM_FusRearPath2VSLK/1  "LM_FusRearPath2VSLK"
  Constant1/1 -> LM_FusRearPath1EMLK/1  "LM_FusRearPath1EMLK"
  Constant/1 -> LM_FusRearPath1VSLK/1  "LM_FusRearPath1VSLK"
